simulink model "task"  (R2024b)
settings: Solver=VariableStepAuto  StartTime=0.0  StopTime=10.0  RelTol=1e-3
settings Model: Creator=muradaliyev  LastModifiedBy=muradaliyev

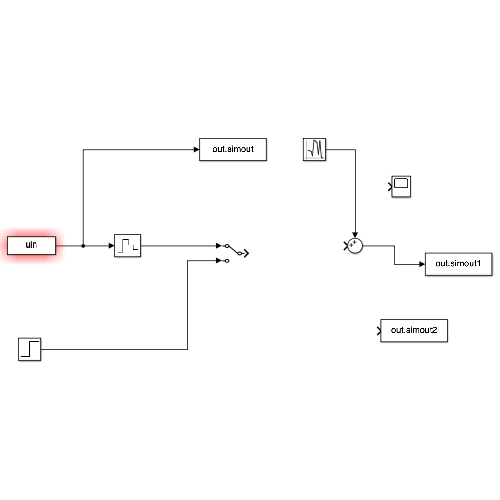
[thumbnail: Simulink's stored preview of the top-level diagram]
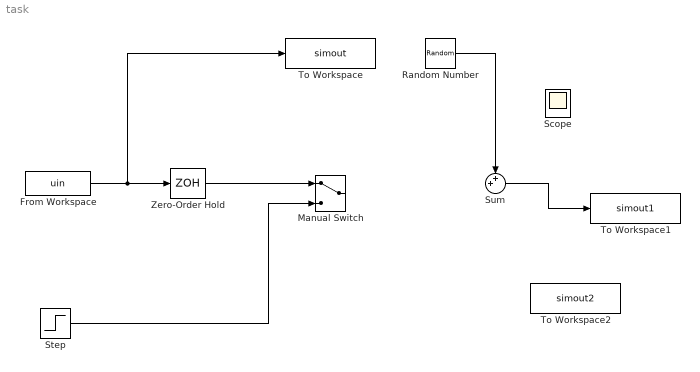
== system task ==
  From Workspace : FromWorkspace  VariableName=uin
  Manual Switch : ManualSwitch
  Random Number : RandomNumber  SampleTime=0.1
  Scope : Scope
  Step : Step  SampleTime=0
  Sum : Sum  Inputs=++|
  To Workspace : ToWorkspace  VariableName=simout  SaveFormat=Timeseries  SampleTime=-1
  To Workspace1 : ToWorkspace  VariableName=simout1  SaveFormat=Timeseries  SampleTime=-1
  To Workspace2 : ToWorkspace  VariableName=simout2  SaveFormat=Timeseries  SampleTime=-1
  Zero-Order Hold : ZeroOrderHold  SampleTime=-1
  wires:
  From Workspace/1 -> To Workspace/1, Zero-Order Hold/1
  Zero-Order Hold/1 -> Manual Switch/1
  Step/1 -> Manual Switch/2
  Sum/1 -> To Workspace1/1
  Random Number/1 -> Sum/1
